simulink model "pathPlanningBicycleSimulinkModel"  (R2020a)
settings: Solver=VariableStepAuto  StartTime=0.0  StopTime=10000  RelTol=1e-3
PostLoadFcn:
  | set_param(gcs, 'ForceConsistencyChecking', 'off');
model workspace (MAT data in the model file):
  Sig = Simulink.Signal
  Sig.DataType = 'auto'
  Sig.Dimensions = -1
  Sig.DimensionsMode = 'auto'
  Sig.Complexity = 'auto'
  Sig.SampleTime = -1
  Sig.SamplingMode = 'auto'
undefined symbols (not defined in the file): goalLoc, QCarMap, startLoc
libraries: robotmobilelib x1, robotalgslib x1
settings Model: OrderedModelArguments=off  Creator=The MathWorks, Inc.  LastModifiedBy=guyot
settings DebuggingCC: SymbolicDimsDataTypeCodeGenerationDiagnostic=none

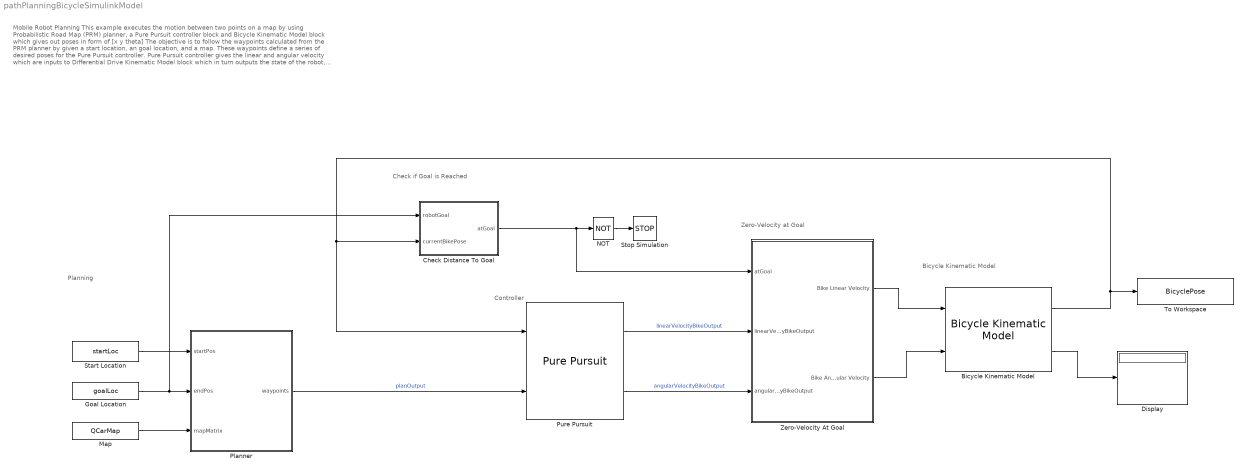
== system pathPlanningBicycleSimulinkModel ==
  note: Check if Goal is Reached
  note: Bicycle Kinematic Model
  note: Controller
  note: Planning
  note: Mobile Robot Planning
      | This example executes the motion between two points on a map by using Probabilistic Road Map (PRM) planner, a Pure Pursuit controller block and Bicycle Kinematic Model block which gives out poses in form of [x y theta]
      |
      | The objective is to follow the waypoints calculated from the PRM planner by given a start location, an goal location, and a map. These waypoints define a series of desired poses for the Pure Pursuit controller.
      |
      | Pure Pursuit controller gives the linear and angular velocity which are inputs to Differential Drive Kinematic Model block which in turn outputs the state of the robot, and its time derivative. To check whether robot has reached its goal state, the distance of the robot from the goal location is measured during simulation, and if this is within a certain threshold, the robot is said to have reached the goal.
      |
      | © Copyright 2019 The MathWorks, Inc.
  note: Zero-Velocity at Goal
  Bicycle Kinematic Model : robotmobilelib/Bicycle Kinematic Model  VehicleInputs=Vehicle Speed & Heading Angular Velocity  WheelBase=0.5  VehicleSpeedRange=[-1 1]  MaxSteeringAngle=pi/3  InitialState=initialBicycle  SimulateUsing=Interpreted execution
      settings: SourceProductBaseCode=RO
  Check Distance To Goal : Subsystem
  Display : Display
  Goal Location : Constant  Value=goalLoc
  Map : Constant  Value=QCarMap
  NOT : Logic  Operator=NOT  IconShape=distinctive  AllPortsSameDT=off  OutDataTypeStr=boolean
  Planner : MATLAB Function  TreatAsAtomicUnit=on
  Pure Pursuit : robotalgslib/Pure Pursuit  DesiredLinearVelocity=0.1  MaxAngularVelocity=1.0  LookaheadDistance=0.5  TargetDirPort=off  SimulateUsing=Code generation
  Start Location : Constant  Value=startLoc
  Stop Simulation : Stop
  To Workspace : ToWorkspace  VariableName=BicyclePose  SampleTime=-1
  Zero-Velocity At Goal : Subsystem
  wires:
  Check Distance To Goal/1(atGoal) -> Zero-Velocity At Goal/1(atGoal), NOT/1
  Pure Pursuit/1 -> Zero-Velocity At Goal/2(linearVelocityBikeOutput)  "linearVelocityBikeOutput"
  Planner/1(waypoints) -> Pure Pursuit/2  "planOutput"
  Pure Pursuit/2 -> Zero-Velocity At Goal/3(angularVelocityBikeOutput)  "angularVelocityBikeOutput"
  Start Location/1 -> Planner/1(startPos)
  Goal Location/1 -> Check Distance To Goal/1(robotGoal), Planner/2(endPos)
  Map/1 -> Planner/3(mapMatrix)
  Bicycle Kinematic Model/1 -> Check Distance To Goal/2(currentBikePose), Pure Pursuit/1, To Workspace/1
  NOT/1 -> Stop Simulation/1
  Zero-Velocity At Goal/1(Bike Linear Velocity) -> Bicycle Kinematic Model/1
  Zero-Velocity At Goal/2(Bike Angular Velocity) -> Bicycle Kinematic Model/2
  Bicycle Kinematic Model/2 -> Display/1

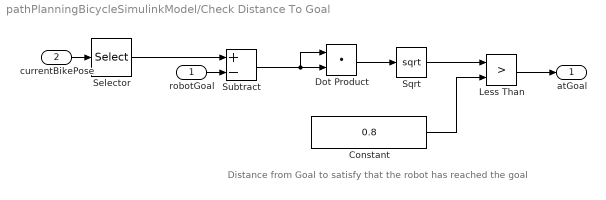
== system pathPlanningBicycleSimulinkModel/Check Distance To Goal ==
  note: Distance from Goal to satisfy that the robot has reached the goal
  robotGoal : Inport
  currentBikePose : Inport  Port=2
  Constant : Constant  Value=0.8
  Dot Product : DotProduct  InputSameDT=on  OutDataTypeStr=Inherit: Inherit via internal rule
  Less Than : RelationalOperator  Operator=>  OutDataTypeStr=boolean  RndMeth=Simplest
  Selector : Selector  InputPortWidth=3  IndexOptions=Index vector (dialog)  Indices=[1 2]  OutputSizes=1
  Sqrt : Sqrt  SaturateOnIntegerOverflow=on
  Subtract : Sum  Inputs=+-
  atGoal : Outport
  wires:
  robotGoal/1 -> Subtract/2
  Dot Product/1 -> Sqrt/1
  Constant/1 -> Less Than/2
  currentBikePose/1 -> Selector/1
  Less Than/1 -> atGoal/1
  Sqrt/1 -> Less Than/1
  Subtract/1 -> Dot Product/1, Dot Product/2
  Selector/1 -> Subtract/1

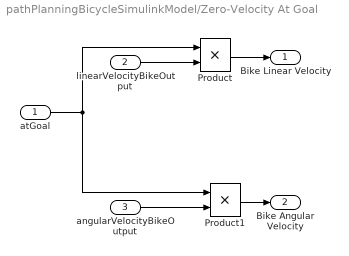
== system pathPlanningBicycleSimulinkModel/Zero-Velocity At Goal ==
  atGoal : Inport
  linearVelocityBikeOutput : Inport  Port=2
  angularVelocityBikeOutput : Inport  Port=3
  Product : Product
  Product1 : Product
  Bike Linear Velocity : Outport  OutDataTypeStr=double
  Bike Angular Velocity : Outport  Port=2  OutDataTypeStr=double
  wires:
  atGoal/1 -> Product1/1, Product/1
  angularVelocityBikeOutput/1 -> Product1/2
  linearVelocityBikeOutput/1 -> Product/2
  Product/1 -> Bike Linear Velocity/1
  Product1/1 -> Bike Angular Velocity/1

== matlab function pathPlanningBicycleSimulinkModel/Planner ==
  settings: updateMethod=DISCRETE
  data: startPos input size=[1 2]; endPos input size=[1 2]; waypoints output size=[100 2]; mapMatrix input
function waypoints = planning(startPos, endPos, mapMatrix)

persistent waypointsInternal
persistent prevStartPos
persistent prevEndPos

% Set constant parameters
maxNumNodes = 100;

% Initialize persistent variables that are used downstream
if isempty(prevStartPos)
    prevStartPos = startPos;
end

if isempty(prevEndPos)
    prevEndPos = endPos;
end

isNewPath = (~isequal(prevStartPos, startPos) || ~isequal(prevEndPos, endPos));

if isempty(waypointsInternal) || isNewPath
    % Two conditions in which waypoints must be set: they are not yet
    % initialized, or they are initialized, but the current start and end
    % do not match those used to generate the previous set of waypoints
    [waypointsInternal] = planPath(mapMatrix, maxNumNodes, startPos, endPos);
end

% Update the outputs
waypoints = waypointsInternal;

% Update the persistent variables that indicate previous state
prevStartPos = startPos;
prevEndPos = endPos;

%% Helper Function

function wayPoints = planPath(mapMatrix, maxNodes, startPos, endPos)
    
    % Create a probabilistic roadmap
    map = binaryOccupancyMap(mapMatrix);
    prm = mobileRobotPRM(map, maxNodes);
    
    % Find a path between two points
    xy = findpath(prm, startPos(:)', endPos(:)');
    wayPoints = repmat(endPos(:)', maxNodes, 1);
    
    % Number of nodes that are actually used
    numNodes = length(xy);
    wayPoints(1:numNodes,:) = xy;    

end

end
